simulink model "PCS_Simulation_Enviroment"  (R2020a)
settings: Solver=VariableStepAuto  StartTime=0.0  StopTime=10.0  RelTol=1e-3
settings Model: DataDictionary=PCS_Simulation_EnviromentDD.sldd  OrderedModelArguments=off  Creator=ykamatan  LastModifiedBy=ykamatan

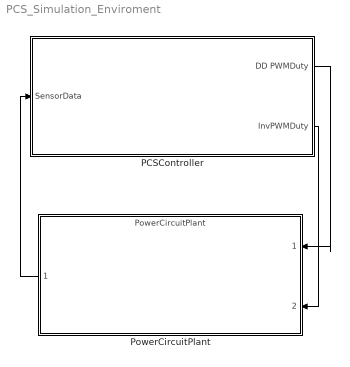
== system PCS_Simulation_Enviroment ==
  PCSController : Subsystem
      settings: PortSchema="{\"entries\":[{\"content\":{\"headerSize\":26,\"margin\":15,\"minimumSpacing\":25,\"sides\":[{\"content\":{\"connectorIds\":[\"In1\"]},\"type\":\"ConnectorPlacement.EquallySpacedRectSide\",\"uuid\":\"9796e929-be55-42a1-ab24-30bc555d00ea\"},{\"content\":{\"connectorIds\":[\"Out1\",\"Out2\"],\"side\":\"RIGHT\"},\"type\":\"ConnectorPlacement.EquallySpacedRectSide\",\"uuid\":\"a0e2ec08-d94c-41f4-8573-1de63b77b3ef\"},{\"content\":{\"connectorIds\":[],\"side\":\"TOP\"},\"type\":\"ConnectorPlacement.EquallySpacedRectSide\",\"uuid\":\"010860e1-918e-4c20-935d-9b338540c304\"},{\"content\":{\"connectorIds\":[],\"side\":\"BOTTOM\"},\"type\":\"ConnectorPlacement.EquallySpacedRectSide\",\"uuid\":\"85090423-0fba-4bdf-9f03-055a85734b91\"}]},\"type\":\"ConnectorPlacement.EquallySpacedConnector\",\"uuid\":\"a2fa6d8f-e467-48a9-a7e8-bd9847d095d5\"}],\"packageUris\":[\"http://schema.mathworks.com/mf0/Connector/19700101\"],\"version\":\"1.0\"}"
  PowerCircuitPlant : ModelReference  ModelNameDialog=PowerCircuitPlant  SimulationMode=Normal  ModelReferenceVersion=1.6
      settings: PortSchema="{\"entries\":[{\"content\":{\"headerSize\":38,\"margin\":15,\"minimumSpacing\":25,\"sides\":[{\"content\":{\"connectorIds\":[\"Out1\"]},\"type\":\"ConnectorPlacement.EquallySpacedRectSide\",\"uuid\":\"9796e929-be55-42a1-ab24-30bc555d00ea\"},{\"content\":{\"connectorIds\":[\"In1\",\"In2\"],\"side\":\"RIGHT\"},\"type\":\"ConnectorPlacement.EquallySpacedRectSide\",\"uuid\":\"a0e2ec08-d94c-41f4-8573-1de63b77b3ef\"},{\"content\":{\"connectorIds\":[],\"side\":\"TOP\"},\"type\":\"ConnectorPlacement.EquallySpacedRectSide\",\"uuid\":\"010860e1-918e-4c20-935d-9b338540c304\"}]},\"type\":\"ConnectorPlacement.EquallySpacedConnector\",\"uuid\":\"a2fa6d8f-e467-48a9-a7e8-bd9847d095d5\"}],\"packageUris\":[\"http://schema.mathworks.com/mf0/Connector/19700101\"],\"version\":\"1.0\"}"
  wires:
  PowerCircuitPlant/1 -> PCSController/1(SensorData)
  PCSController/1(DD PWMDuty) -> PowerCircuitPlant/1
  PCSController/2(InvPWMDuty) -> PowerCircuitPlant/2

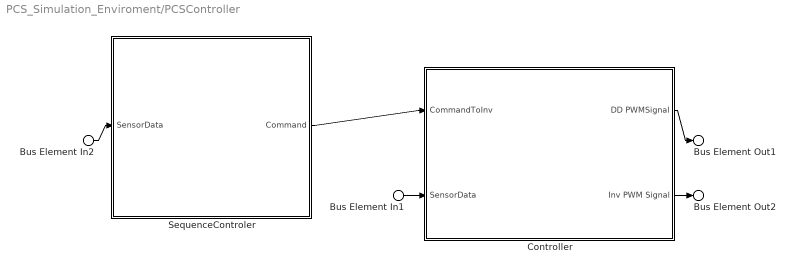
== system PCS_Simulation_Enviroment/PCSController ==
  Bus Element In1 : Inport  PortName=SensorData
  Bus Element In2 : Inport  PortName=SensorData
  Controller : Subsystem
      settings: PortSchema="{\"entries\":[{\"content\":{\"headerSize\":26,\"margin\":15,\"minimumSpacing\":25,\"sides\":[{\"content\":{\"connectorIds\":[\"In1\",\"In2\"]},\"type\":\"ConnectorPlacement.EquallySpacedRectSide\",\"uuid\":\"6d5a3475-51d4-4fed-a4a1-1c259683418a\"},{\"content\":{\"connectorIds\":[\"Out1\",\"Out2\"],\"side\":\"RIGHT\"},\"type\":\"ConnectorPlacement.EquallySpacedRectSide\",\"uuid\":\"687f9b37-d781-487a-8ccc-4d9d98ae2b03\"},{\"content\":{\"connectorIds\":[],\"side\":\"TOP\"},\"type\":\"ConnectorPlacement.EquallySpacedRectSide\",\"uuid\":\"358978ee-aad2-4ede-9f11-36687296ed36\"}]},\"type\":\"ConnectorPlacement.EquallySpacedConnector\",\"uuid\":\"41535ad0-fa46-427f-b800-3adbc14a3515\"}],\"packageUris\":[\"http://schema.mathworks.com/mf0/Connector/19700101\"],\"version\":\"1.0\"}"
  SequenceControler : Subsystem
      settings: PortSchema="{\"entries\":[{\"content\":{\"headerSize\":26,\"margin\":15,\"minimumSpacing\":25,\"sides\":[{\"content\":{\"connectorIds\":[\"In1\"]},\"type\":\"ConnectorPlacement.EquallySpacedRectSide\",\"uuid\":\"9796e929-be55-42a1-ab24-30bc555d00ea\"},{\"content\":{\"connectorIds\":[\"Out1\"],\"side\":\"RIGHT\"},\"type\":\"ConnectorPlacement.EquallySpacedRectSide\",\"uuid\":\"a0e2ec08-d94c-41f4-8573-1de63b77b3ef\"},{\"content\":{\"connectorIds\":[],\"side\":\"TOP\"},\"type\":\"ConnectorPlacement.EquallySpacedRectSide\",\"uuid\":\"010860e1-918e-4c20-935d-9b338540c304\"},{\"content\":{\"connectorIds\":[],\"side\":\"BOTTOM\"},\"type\":\"ConnectorPlacement.EquallySpacedRectSide\",\"uuid\":\"1178fdb8-ac02-4f81-8387-b01af1048b4e\"}]},\"type\":\"ConnectorPlacement.EquallySpacedConnector\",\"uuid\":\"a2fa6d8f-e467-48a9-a7e8-bd9847d095d5\"}],\"packageUris\":[\"http://schema.mathworks.com/mf0/Connector/19700101\"],\"version\":\"1.0\"}"
  Bus Element Out1 : Outport  PortName=DD PWMDuty
  Bus Element Out2 : Outport  Port=2  PortName=InvPWMDuty
  wires:
  SequenceControler/1(Command) -> Controller/1(CommandToInv)
  Bus Element In1/1 -> Controller/2(SensorData)
  Bus Element In2/1 -> SequenceControler/1(SensorData)
  Controller/1(DD PWMSignal) -> Bus Element Out1/1
  Controller/2(Inv PWM Signal) -> Bus Element Out2/1

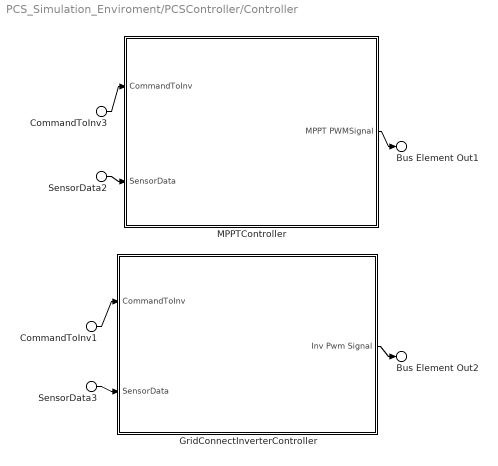
== system PCS_Simulation_Enviroment/PCSController/Controller ==
  CommandToInv1 : Inport  PortName=CommandToInv
  CommandToInv3 : Inport  PortName=CommandToInv
  SensorData2 : Inport  Port=2  PortName=SensorData
  SensorData3 : Inport  Port=2  PortName=SensorData
  GridConnectInverterController : Subsystem
      settings: PortSchema="{\"entries\":[{\"content\":{\"headerSize\":26,\"margin\":15,\"minimumSpacing\":25,\"sides\":[{\"content\":{\"connectorIds\":[\"In1\",\"In2\"]},\"type\":\"ConnectorPlacement.EquallySpacedRectSide\",\"uuid\":\"9796e929-be55-42a1-ab24-30bc555d00ea\"},{\"content\":{\"connectorIds\":[\"Out1\"],\"side\":\"RIGHT\"},\"type\":\"ConnectorPlacement.EquallySpacedRectSide\",\"uuid\":\"a0e2ec08-d94c-41f4-8573-1de63b77b3ef\"},{\"content\":{\"connectorIds\":[],\"side\":\"TOP\"},\"type\":\"ConnectorPlacement.EquallySpacedRectSide\",\"uuid\":\"010860e1-918e-4c20-935d-9b338540c304\"}]},\"type\":\"ConnectorPlacement.EquallySpacedConnector\",\"uuid\":\"a2fa6d8f-e467-48a9-a7e8-bd9847d095d5\"}],\"packageUris\":[\"http://schema.mathworks.com/mf0/Connector/19700101\"],\"version\":\"1.0\"}"
  MPPTController : Subsystem
      settings: PortSchema="{\"entries\":[{\"content\":{\"headerSize\":26,\"margin\":15,\"minimumSpacing\":25,\"sides\":[{\"content\":{\"connectorIds\":[\"In1\",\"In2\"]},\"type\":\"ConnectorPlacement.EquallySpacedRectSide\",\"uuid\":\"9796e929-be55-42a1-ab24-30bc555d00ea\"},{\"content\":{\"connectorIds\":[\"Out1\"],\"side\":\"RIGHT\"},\"type\":\"ConnectorPlacement.EquallySpacedRectSide\",\"uuid\":\"a0e2ec08-d94c-41f4-8573-1de63b77b3ef\"},{\"content\":{\"connectorIds\":[],\"side\":\"TOP\"},\"type\":\"ConnectorPlacement.EquallySpacedRectSide\",\"uuid\":\"010860e1-918e-4c20-935d-9b338540c304\"}]},\"type\":\"ConnectorPlacement.EquallySpacedConnector\",\"uuid\":\"a2fa6d8f-e467-48a9-a7e8-bd9847d095d5\"}],\"packageUris\":[\"http://schema.mathworks.com/mf0/Connector/19700101\"],\"version\":\"1.0\"}"
  Bus Element Out1 : Outport  PortName=DD PWMSignal
  Bus Element Out2 : Outport  Port=2  PortName=Inv PWM Signal
  wires:
  SensorData3/1 -> GridConnectInverterController/2(SensorData)
  SensorData2/1 -> MPPTController/2(SensorData)
  CommandToInv1/1 -> GridConnectInverterController/1(CommandToInv)
  CommandToInv3/1 -> MPPTController/1(CommandToInv)
  MPPTController/1(MPPT PWMSignal) -> Bus Element Out1/1
  GridConnectInverterController/1(Inv Pwm Signal) -> Bus Element Out2/1

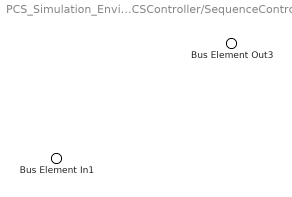
== system PCS_Simulation_Enviroment/PCSController/SequenceControler ==
  Bus Element In1 : Inport  PortName=SensorData
  Bus Element Out3 : Outport  PortName=Command

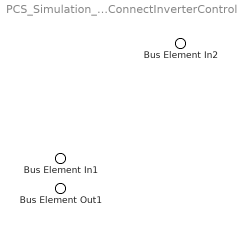
== system PCS_Simulation_Enviroment/PCSController/Controller/GridConnectInverterController ==
  Bus Element In2 : Inport  PortName=CommandToInv
  Bus Element In1 : Inport  Port=2  PortName=SensorData
  Bus Element Out1 : Outport  PortName=Inv Pwm Signal

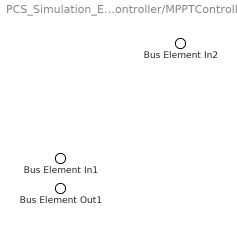
== system PCS_Simulation_Enviroment/PCSController/Controller/MPPTController ==
  Bus Element In2 : Inport  PortName=CommandToInv
  Bus Element In1 : Inport  Port=2  PortName=SensorData
  Bus Element Out1 : Outport  PortName=MPPT PWMSignal
